simulink model "Sistema"  (R2023a)
settings: Solver=ode15s  StartTime=0.0  StopTime=10.0  MaxStep=1E-3  RelTol=1e-3
libraries: fl_lib x18, nesl_utility x9, ee_lib x3, slpidlib x2
settings Model: LastModifiedBy=alan_25
settings DataIOCC: SaveFormat=Array  ReturnWorkspaceOutputs=off  TimeSaveName=t
settings DebuggingCC: AlgebraicLoopMsg=none  ArtificialAlgebraicLoopMsg=none  ModelReferenceExtraNoncontSigs=none  OperatingPointInterfaceChecksumMismatchMsg=none
settings RTWCC: GPUComputeCapability=5.0

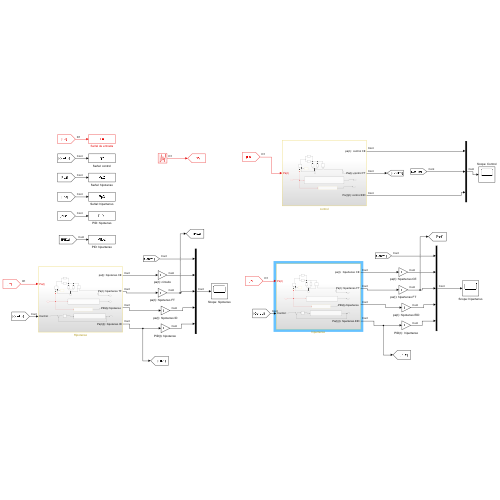
[thumbnail: Simulink's stored preview of the top-level diagram]
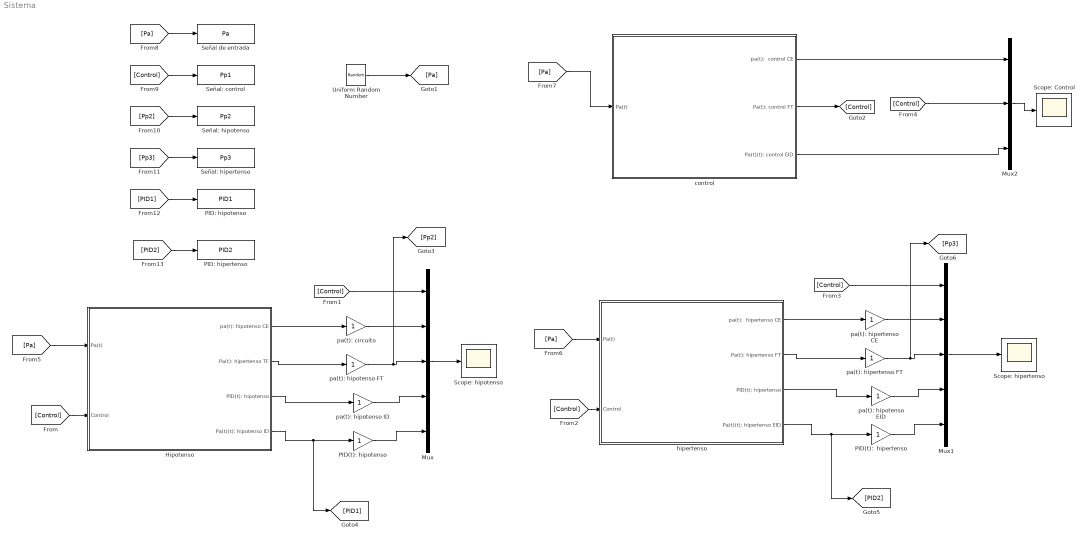
== system Sistema ==
  Hipotenso : Subsystem
  Mux : Mux  Inputs=5
  Mux1 : Mux  Inputs=5
  Mux2 : Mux  Inputs=3
  PID(t):  hipertenso : Gain
  "PID(t): hipotenso " : Gain
  PID: hipertenso : ToWorkspace  VariableName=PID2  SampleTime=-1
  PID: hipotenso : ToWorkspace  VariableName=PID1  SampleTime=-1
  Scope: Control : Scope
  Scope: hipertenso : Scope
  Scope: hipotenso : Scope
  Señal de entrada : ToWorkspace  VariableName=Pa  SampleTime=-1
  Señal: control : ToWorkspace  VariableName=Pp1  SampleTime=-1
  Señal: hipertenso : ToWorkspace  VariableName=Pp3  SampleTime=-1
  Señal: hipotenso : ToWorkspace  VariableName=Pp2  SampleTime=-1
  Uniform Random Number : UniformRandomNumber  Minimum=-0.2  Seed=106  SampleTime=0.5
  control : Subsystem
  hipertenso : Subsystem
  pa(t): circuito : Gain
  pa(t): hipertenso CE : Gain
  pa(t): hipertenso FT : Gain
  pa(t): hipotenso EID : Gain
  pa(t): hipotenso FT : Gain
  pa(t): hipotenso ID : Gain
  wires:
  Mux/1 -> Scope: hipotenso/1
  [Control] -> Hipotenso/2(Control)
  [Control] -> Mux/1
  Hipotenso/1(pa(t): hipotenso CE) -> pa(t): circuito/1
  pa(t): circuito/1 -> Mux/2
  "PID(t): hipotenso "/1 -> Mux/5
  Hipotenso/4(Pa(t)(t): hipotenso ID) -> [PID1], "PID(t): hipotenso "/1
  Hipotenso/3("PID(t): hipotenso ") -> pa(t): hipotenso ID/1
  pa(t): hipotenso ID/1 -> Mux/4
  pa(t): hipotenso FT/1 -> [Pp2], Mux/3
  Hipotenso/2(Pa(t): hipertenso TF) -> pa(t): hipotenso FT/1
  hipertenso/1(pa(t):  hipertenso CE) -> pa(t): hipertenso CE/1
  pa(t): hipertenso FT/1 -> [Pp3], Mux1/3
  hipertenso/2(Pa(t): hipertenso FT) -> pa(t): hipertenso FT/1
  pa(t): hipotenso EID/1 -> Mux1/4
  [Control] -> hipertenso/2(Control)
  Mux1/1 -> Scope: hipertenso/1
  [Control] -> Mux1/1
  pa(t): hipertenso CE/1 -> Mux1/2
  hipertenso/4(Pa(t)(t): hipertenso EID) -> [PID2], PID(t):  hipertenso/1
  PID(t):  hipertenso/1 -> Mux1/5
  hipertenso/3("PID(t): hipertenso ") -> pa(t): hipotenso EID/1
  Uniform Random Number/1 -> [Pa]
  [Pa] -> Hipotenso/1(Pa(t))
  [Pa] -> hipertenso/1(Pa(t))
  Mux2/1 -> Scope: Control/1
  [Pa] -> control/1(Pa(t))
  control/2(Pa(t): control FT) -> [Control]
  [Control] -> Mux2/2
  control/1(pa(t):  control CE) -> Mux2/1
  control/3(Pa(t)(t): control EID) -> Mux2/3
  [Pa] -> Señal de entrada/1
  [Control] -> Señal: control/1
  [Pp2] -> Señal: hipotenso/1
  [Pp3] -> Señal: hipertenso/1
  [PID1] -> PID: hipotenso/1
  [PID2] -> PID: hipertenso/1

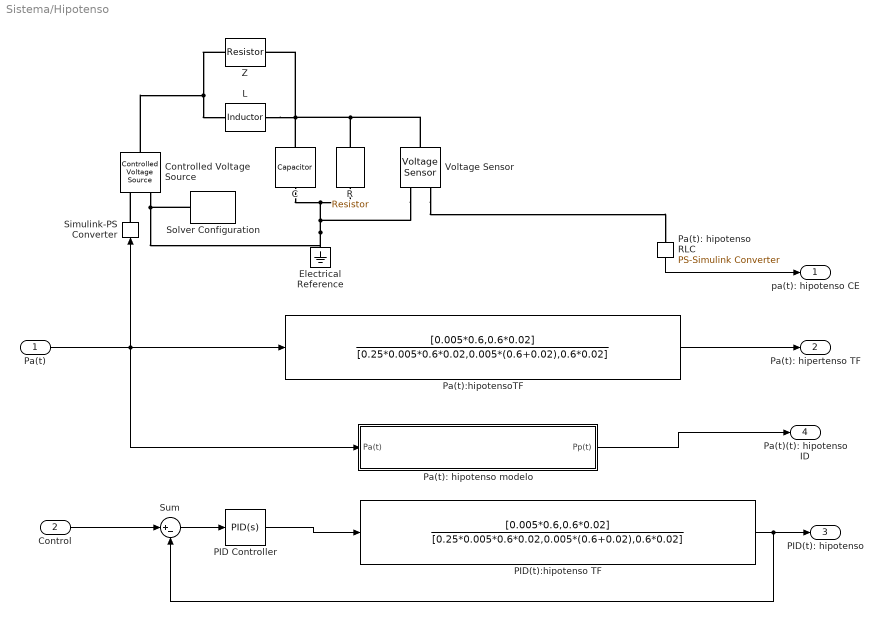
== system Sistema/Hipotenso ==
  Pa(t) : Inport
  Control : Inport  Port=2
  C : fl_lib/Electrical/Electrical Elements/Capacitor  c=0.25 F  r=1e-6 Ohm  g=0 1/Ohm  i_specify=off  i_priority=None  i=0 A  i_nominal_specify=off  i_nominal_unit=A  i_nominal_value=1  v_specify=off  v_priority=None  v=0 V  v_nominal_specify=off  v_nominal_unit=V  v_nominal_value=1  vc_specify=off  vc_priority=High  vc=0 V  vc_nominal_specify=off  vc_nominal_unit=V  vc_nominal_value=1
  Controlled Voltage Source : fl_lib/Electrical/Electrical Sources/Controlled Voltage Source
  Electrical Reference : fl_lib/Electrical/Electrical Elements/Electrical Reference
  L : ee_lib/Passive/Inductor  l=0.005 H  enable_L_tol=ee.enum.toleranceApplication.none  L_tol=20  tol_distribution=ee.enum.toleranceDistribution.uniform  nSigma=4  r=0 Ohm  g=1e-9 1/Ohm  enable_operating_limits=ee.enum.enable.no  operating_limit_action=ee.enum.passive.reportOpLim.warn  max_working_current=1 A  power_rating=1 W  enable_faults=ee.enum.enable.no  fault_action=simscape.enum.assert.action.none  lambdaPercent=50  k_faulted=0.9999  turnsShort=ee.enum.passive.inductor.turnsShortOption.no  openCct=ee.enum.enable.no  groundShort=ee.enum.passive.inductor.groundShortOption.no  groundShortG=0 1/Ohm  tau_fault=1e-3 s  fault_trigger=ee.enum.faults.faultTrigger.temporal  t_fault=1 s  max_permissible_voltage=100 V  n_fail_on_voltage=1  max_permissible_current=1 A  t_fail_on_current=1 s  i_L_specify=off  i_L_priority=High  i_L=0 A  i_L_nominal_specify=off  i_L_nominal_unit=A  i_L_nominal_value=1
  PID Controller : slpidlib/PID Controller  Controller=PID  Form=Parallel  TimeDomain=Continuous-time  UseExternalTs=off  SampleTime=-1  IntegratorMethod=Forward Euler  FilterMethod=Forward Euler  ControllerParametersSource=internal  P=1.49397900518606  I=352.000659394334  UseKiTs=off  D=0.00049119206492278  N=536.918505743178  UseFilter=on  TunerSelectOption=Transfer Function Based (PID Tuner App)  InitialConditionSource=internal  InitialConditionForIntegrator=0  InitialConditionForFilter=0  DifferentiatorICPrevScaledInput=0  ExternalReset=none  TrackingMode=off  Kt=1  LimitOutput=off  SatLimitsSource=internal  UpperSaturationLimit=inf  LowerSaturationLimit=-inf  LinearizeAsGain=on  AntiWindupMode=none  Kb=1  LimitIntegrator=off  UpperIntegratorSaturationLimit=inf  LowerIntegratorSaturationLimit=-inf  POutMin=[]  POutMax=[]  IOutMin=[]  IOutMax=[]  DOutMin=[]  DOutMax=[]  NOutMin=[]  NOutMax=[]  SumOutMin=[]  SumOutMax=[]  SaturationOutMin=[]  SaturationOutMax=[]  PParamMin=[]  PParamMax=[]  IParamMin=[]  IParamMax=[]  DParamMin=[]  DParamMax=[]  NParamMin=[]  NParamMax=[]  KbParamMin=[]  KbParamMax=[]  KtParamMin=[]  KtParamMax=[]  KbOutMin=[]  KbOutMax=[]  KtOutMin=[]  KtOutMax=[]  IntegratorOutMin=[]  IntegratorOutMax=[]  FilterOutMin=[]  FilterOutMax=[]  SumI1OutMin=[]  SumI1OutMax=[]  SumI2OutMin=[]  SumI2OutMax=[]  SumI3OutMin=[]  SumI3OutMax=[]  SumI4OutMin=[]  SumI4OutMax=[]  SumDOutMin=[]  SumDOutMax=[]  DifferentiatorOutMin=[]  DifferentiatorOutMax=[]  FilterDiffOutCoefMin=[]  FilterDiffOutCoefMax=[]  ReciprocalOutMin=[]  ReciprocalOutMax=[]  SumDenOutMin=[]  SumDenOutMax=[]  SumNumOutMin=[]  SumNumOutMax=[]  DivideOutMin=[]  DivideOutMax=[]  UdiffTsProdOutMin=[]  UdiffTsProdOutMax=[]  NTsProdOutMin=[]  NTsProdOutMax=[]  UintegralTsProdOutMin=[]  UintegralTsProdOutMax=[]  UngainTsProdOutMin=[]  UngainTsProdOutMax=[]  ClampingZeroOutDataTypeStr=Inherit: Inherit via back propagation  ClampingZeroOutMin=[]  ClampingZeroOutMax=[]  FilterDenConstantOutDataTypeStr=Inherit: Inherit via back propagation  FilterDenConstantOutMin=[]  FilterDenConstantOutMax=[]  PCopyOutDataTypeStr=Inherit: Inherit via back propagation  PCopyOutMin=[]  PCopyOutMax=[]  NCopyOutDataTypeStr=Inherit: Inherit via back propagation  NCopyOutMin=[]  NCopyOutMax=[]  IntegratorContinuousStateAttributes=''  IntegratorStateMustResolveToSignalObject=off  IntegratorRTWStateStorageClass=Auto  FilterContinuousStateAttributes=''  FilterStateMustResolveToSignalObject=off  FilterRTWStateStorageClass=Auto  ParallelPVariant=InternalParameters  IdealPVariant=Disabled  IVariant=InternalParameters  DVariant=InternalParameters  IntegratorVariant=Continuous  SatVariant=Disabled  AWVariant=Passthrough  PCopyVariant=Disabled  TRVariant=Disabled  FdbkBlocksVariant=Forward  IdealPFdbkVariant=Disabled  SatFdbkVariant=Disabled  DerivativeFilterVariant=ContFilter  NVariant=InternalParameters  NCopyVariant=Disabled  FilterICVariant=InternalICsFilter  IntegratorICVariant=InternalICs  ExternalResetVariant=Disabled  TRSumVariant=Passthrough  SumFdbkVariant=Disabled  SumVariant=Sum_PID  TsampFilterVariant=InternalTs  TsampNgainVariant=Passthrough  TsampIntegralVariant=Disabled_SignalSpec  ExternalSaturationOutDataTypeStr=Inherit: Same as second input
  PID(t):hipotenso TF : TransferFcn  Numerator=[0.005*0.6,0.6*0.02]  Denominator=[0.25*0.005*0.6*0.02,0.005*(0.6+0.02),0.6*0.02]
  Pa(t): hipotenso RLC : nesl_utility/PS-Simulink Converter  PhysicalDomain=network_engine_domain  SubClassName=ps_output  LeftPortType=input  RightPortType=output  PseudoPeriodic=off  Frequencies=[]  VectorFormat=1-D array  Unit=inherit  AffineConversion=off
  Pa(t): hipotenso modelo : Subsystem  TreatAsAtomicUnit=on
  Pa(t):hipotensoTF : TransferFcn  Numerator=[0.005*0.6,0.6*0.02]  Denominator=[0.25*0.005*0.6*0.02,0.005*(0.6+0.02),0.6*0.02]
  R : fl_lib/Electrical/Electrical Elements/Resistor  R=0.6 Ohm  i_specify=off  i_priority=None  i=0 A  i_nominal_specify=off  i_nominal_unit=A  i_nominal_value=1  v_specify=off  v_priority=None  v=0 V  v_nominal_specify=off  v_nominal_unit=V  v_nominal_value=1
  Simulink-PS Converter : nesl_utility/Simulink-PS Converter  PhysicalDomain=network_engine_domain  SubClassName=ps_input  LeftPortType=input  RightPortType=output  PseudoPeriodic=off  Frequencies=[]  NoiseDistribution=none  NoiseParameters=[]  Unit=1  AffineConversion=off  FilteringAndDerivatives=provide  SimscapeFilterOrder=1  InputFilterTimeConstant=0.001  UdotUserProvided=0
  Solver Configuration : nesl_utility/Solver Configuration  PhysicalDomain=network_engine_domain  SubClassName=solver  LeftPortType=input  RightPortType=generic  Tones=[]  Harmonics=[]  SimulateNoise=off  Profile=off  UseLocalSampling=off  EnableSwitchedLinearOptims=on  FrequencyDomain=off  UseCCode=off  RelTol=0.001  AbsTol=0.001  MinStep=1e-09  ToWorkspace=off  RevertToSquareIcSolve=off  NumHomotopyIterations=100  PhasorMode=off  PhasorModeNumHarmonics=1  ConsistencySolver=NEWTON_XTOL_AFTER_FTOL  IndexReductionMethod=DerivativeReplacement  DoDC=off  ResidualTolerance=1e-09  ConsistencyTolSource=GLOBAL  ConsistencyAbsTol=0.001  ConsistencyRelTol=0.001  ConsistencyTolFactor=0.001  UseLocalSolver=off  LocalSolverChoice=NE_BACKWARD_EULER_ADVANCER  ResolveIndetEquations=on  FunctionEvalNumThread=1  LocalSolverSampleTime=0.001  DoFixedCost=off  MaxNonlinIter=3  MaxModeIter=2  ComputeImpulses=off  ImpulseIterations=2  LinearAlgebra=auto  LinearAlgebraNumThread=0  EquationFormulation=NE_TIME_EF  DelaysMemoryBudget=1024  AutomaticFiltering=on  FilteringTimeConstant=0.001  PartitionStorageMethod=AS_NEEDED  PartitionMemoryBudget=1024  PartitionMethod=ROBUST
  Sum : Sum  Inputs=|+-
  Voltage Sensor : fl_lib/Electrical/Electrical Sensors/Voltage Sensor
  Z : fl_lib/Electrical/Electrical Elements/Resistor  R=0.02 Ohm  i_specify=off  i_priority=None  i=0 A  i_nominal_specify=off  i_nominal_unit=A  i_nominal_value=1  v_specify=off  v_priority=None  v=0 V  v_nominal_specify=off  v_nominal_unit=V  v_nominal_value=1
  pa(t): hipotenso CE : Outport
  Pa(t): hipertenso TF : Outport  Port=2
  "PID(t): hipotenso " : Outport  Port=3
  Pa(t)(t): hipotenso ID : Outport  Port=4
  wires:
  PID(t):hipotenso TF/1 -> "PID(t): hipotenso "/1, Sum/2
  Sum/1 -> PID Controller/1
  PID Controller/1 -> PID(t):hipotenso TF/1
  Pa(t):hipotensoTF/1 -> Pa(t): hipertenso TF/1
  Pa(t): hipotenso RLC/1 -> pa(t): hipotenso CE/1
  Pa(t)/1 -> Pa(t): hipotenso modelo/1(Pa(t)), Pa(t):hipotensoTF/1, Simulink-PS Converter/1
  Control/1 -> Sum/1
  Pa(t): hipotenso modelo/1(Pp(t)) -> Pa(t)(t): hipotenso ID/1
  connections:
  Voltage Sensor/RConn1 -- Pa(t): hipotenso RLC/LConn1
  L/LConn1 -- Voltage Sensor/LConn1 -- R/LConn1 -- C/LConn1 -- Z/RConn1
  Simulink-PS Converter/RConn1 -- Controlled Voltage Source/RConn1
  Z/LConn1 -- Controlled Voltage Source/LConn1 -- L/RConn1
  C/RConn1 -- Voltage Sensor/RConn2 -- Solver Configuration/RConn1 -- Controlled Voltage Source/RConn2 -- Electrical Reference/LConn1 -- R/RConn1

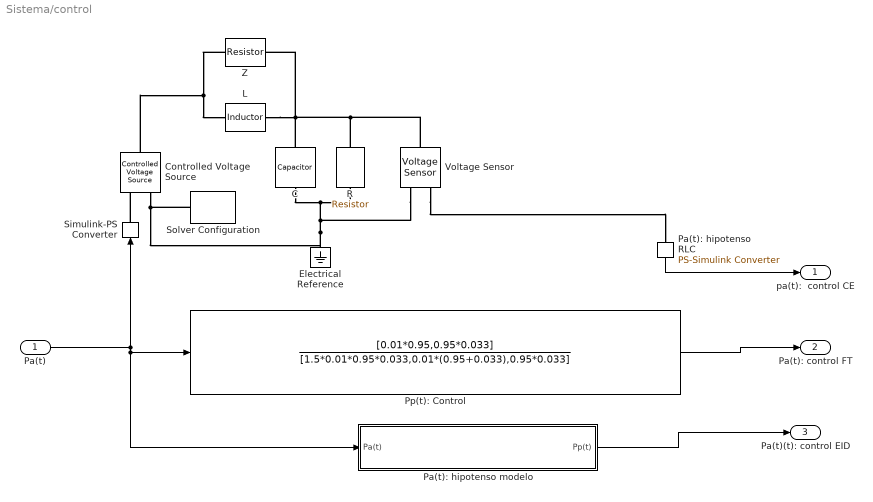
== system Sistema/control ==
  Pa(t) : Inport
  C : fl_lib/Electrical/Electrical Elements/Capacitor  c=1.5 F  r=1e-6 Ohm  g=0 1/Ohm  i_specify=off  i_priority=None  i=0 A  i_nominal_specify=off  i_nominal_unit=A  i_nominal_value=1  v_specify=off  v_priority=None  v=0 V  v_nominal_specify=off  v_nominal_unit=V  v_nominal_value=1  vc_specify=off  vc_priority=High  vc=0 V  vc_nominal_specify=off  vc_nominal_unit=V  vc_nominal_value=1
  Controlled Voltage Source : fl_lib/Electrical/Electrical Sources/Controlled Voltage Source
  Electrical Reference : fl_lib/Electrical/Electrical Elements/Electrical Reference
  L : ee_lib/Passive/Inductor  l=0.01 H  enable_L_tol=ee.enum.toleranceApplication.none  L_tol=20  tol_distribution=ee.enum.toleranceDistribution.uniform  nSigma=4  r=0 Ohm  g=1e-9 1/Ohm  enable_operating_limits=ee.enum.enable.no  operating_limit_action=ee.enum.passive.reportOpLim.warn  max_working_current=1 A  power_rating=1 W  enable_faults=ee.enum.enable.no  fault_action=simscape.enum.assert.action.none  lambdaPercent=50  k_faulted=0.9999  turnsShort=ee.enum.passive.inductor.turnsShortOption.no  openCct=ee.enum.enable.no  groundShort=ee.enum.passive.inductor.groundShortOption.no  groundShortG=0 1/Ohm  tau_fault=1e-3 s  fault_trigger=ee.enum.faults.faultTrigger.temporal  t_fault=1 s  max_permissible_voltage=100 V  n_fail_on_voltage=1  max_permissible_current=1 A  t_fail_on_current=1 s  i_L_specify=off  i_L_priority=High  i_L=0 A  i_L_nominal_specify=off  i_L_nominal_unit=A  i_L_nominal_value=1
  Pa(t): hipotenso RLC : nesl_utility/PS-Simulink Converter  PhysicalDomain=network_engine_domain  SubClassName=ps_output  LeftPortType=input  RightPortType=output  PseudoPeriodic=off  Frequencies=[]  VectorFormat=1-D array  Unit=inherit  AffineConversion=off
  Pa(t): hipotenso modelo : Subsystem  TreatAsAtomicUnit=on
  Pp(t): Control : TransferFcn  Numerator=[0.01*0.95,0.95*0.033]  Denominator=[1.5*0.01*0.95*0.033,0.01*(0.95+0.033),0.95*0.033]
  R : fl_lib/Electrical/Electrical Elements/Resistor  R=0.95 Ohm  i_specify=off  i_priority=None  i=0 A  i_nominal_specify=off  i_nominal_unit=A  i_nominal_value=1  v_specify=off  v_priority=None  v=0 V  v_nominal_specify=off  v_nominal_unit=V  v_nominal_value=1
  Simulink-PS Converter : nesl_utility/Simulink-PS Converter  PhysicalDomain=network_engine_domain  SubClassName=ps_input  LeftPortType=input  RightPortType=output  PseudoPeriodic=off  Frequencies=[]  NoiseDistribution=none  NoiseParameters=[]  Unit=1  AffineConversion=off  FilteringAndDerivatives=provide  SimscapeFilterOrder=1  InputFilterTimeConstant=0.001  UdotUserProvided=0
  Solver Configuration : nesl_utility/Solver Configuration  PhysicalDomain=network_engine_domain  SubClassName=solver  LeftPortType=input  RightPortType=generic  Tones=[]  Harmonics=[]  SimulateNoise=off  Profile=off  UseLocalSampling=off  EnableSwitchedLinearOptims=on  FrequencyDomain=off  UseCCode=off  RelTol=0.001  AbsTol=0.001  MinStep=1e-09  ToWorkspace=off  RevertToSquareIcSolve=off  NumHomotopyIterations=100  PhasorMode=off  PhasorModeNumHarmonics=1  ConsistencySolver=NEWTON_XTOL_AFTER_FTOL  IndexReductionMethod=DerivativeReplacement  DoDC=off  ResidualTolerance=1e-09  ConsistencyTolSource=GLOBAL  ConsistencyAbsTol=0.001  ConsistencyRelTol=0.001  ConsistencyTolFactor=0.001  UseLocalSolver=off  LocalSolverChoice=NE_BACKWARD_EULER_ADVANCER  ResolveIndetEquations=on  FunctionEvalNumThread=1  LocalSolverSampleTime=0.001  DoFixedCost=off  MaxNonlinIter=3  MaxModeIter=2  ComputeImpulses=off  ImpulseIterations=2  LinearAlgebra=auto  LinearAlgebraNumThread=0  EquationFormulation=NE_TIME_EF  DelaysMemoryBudget=1024  AutomaticFiltering=on  FilteringTimeConstant=0.001  PartitionStorageMethod=AS_NEEDED  PartitionMemoryBudget=1024  PartitionMethod=ROBUST
  Voltage Sensor : fl_lib/Electrical/Electrical Sensors/Voltage Sensor
  Z : fl_lib/Electrical/Electrical Elements/Resistor  R=0.033 Ohm  i_specify=off  i_priority=None  i=0 A  i_nominal_specify=off  i_nominal_unit=A  i_nominal_value=1  v_specify=off  v_priority=None  v=0 V  v_nominal_specify=off  v_nominal_unit=V  v_nominal_value=1
  pa(t):  control CE : Outport
  Pa(t): control FT : Outport  Port=2
  Pa(t)(t): control EID : Outport  Port=3
  wires:
  Pa(t): hipotenso RLC/1 -> pa(t):  control CE/1
  Pa(t)/1 -> Pp(t): Control/1, Pa(t): hipotenso modelo/1(Pa(t)), Simulink-PS Converter/1
  Pa(t): hipotenso modelo/1(Pp(t)) -> Pa(t)(t): control EID/1
  Pp(t): Control/1 -> Pa(t): control FT/1
  connections:
  Voltage Sensor/RConn1 -- Pa(t): hipotenso RLC/LConn1
  C/LConn1 -- Z/RConn1 -- L/LConn1 -- Voltage Sensor/LConn1 -- R/LConn1
  Simulink-PS Converter/RConn1 -- Controlled Voltage Source/RConn1
  Z/LConn1 -- L/RConn1 -- Controlled Voltage Source/LConn1
  Electrical Reference/LConn1 -- Voltage Sensor/RConn2 -- C/RConn1 -- R/RConn1 -- Solver Configuration/RConn1 -- Controlled Voltage Source/RConn2

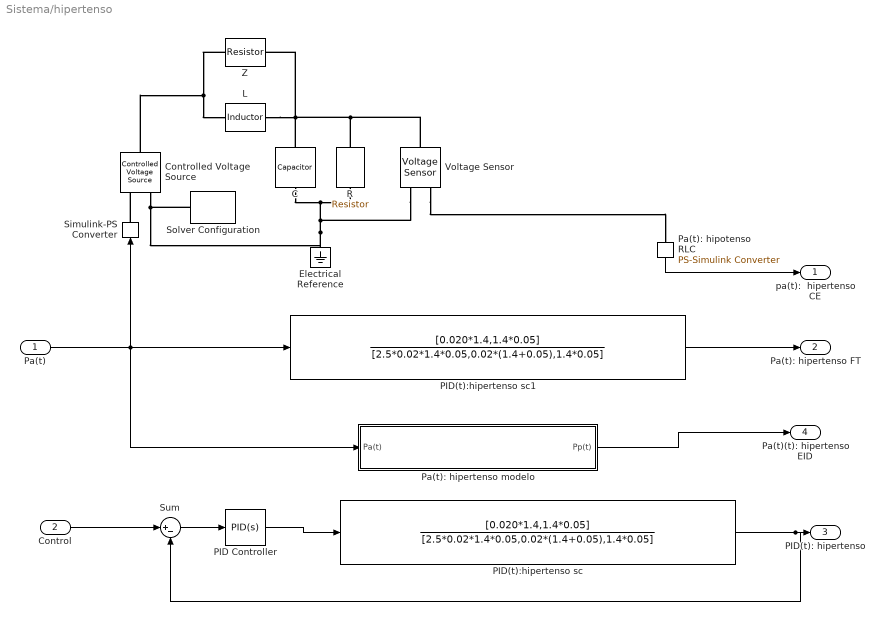
== system Sistema/hipertenso ==
  Pa(t) : Inport
  Control : Inport  Port=2
  C : fl_lib/Electrical/Electrical Elements/Capacitor  c=2.5 F  r=1e-6 Ohm  g=0 1/Ohm  i_specify=off  i_priority=None  i=0 A  i_nominal_specify=off  i_nominal_unit=A  i_nominal_value=1  v_specify=off  v_priority=None  v=0 V  v_nominal_specify=off  v_nominal_unit=V  v_nominal_value=1  vc_specify=off  vc_priority=High  vc=0 V  vc_nominal_specify=off  vc_nominal_unit=V  vc_nominal_value=1
  Controlled Voltage Source : fl_lib/Electrical/Electrical Sources/Controlled Voltage Source
  Electrical Reference : fl_lib/Electrical/Electrical Elements/Electrical Reference
  L : ee_lib/Passive/Inductor  l=0.02 H  enable_L_tol=ee.enum.toleranceApplication.none  L_tol=20  tol_distribution=ee.enum.toleranceDistribution.uniform  nSigma=4  r=0 Ohm  g=1e-9 1/Ohm  enable_operating_limits=ee.enum.enable.no  operating_limit_action=ee.enum.passive.reportOpLim.warn  max_working_current=1 A  power_rating=1 W  enable_faults=ee.enum.enable.no  fault_action=simscape.enum.assert.action.none  lambdaPercent=50  k_faulted=0.9999  turnsShort=ee.enum.passive.inductor.turnsShortOption.no  openCct=ee.enum.enable.no  groundShort=ee.enum.passive.inductor.groundShortOption.no  groundShortG=0 1/Ohm  tau_fault=1e-3 s  fault_trigger=ee.enum.faults.faultTrigger.temporal  t_fault=1 s  max_permissible_voltage=100 V  n_fail_on_voltage=1  max_permissible_current=1 A  t_fail_on_current=1 s  i_L_specify=off  i_L_priority=High  i_L=0 A  i_L_nominal_specify=off  i_L_nominal_unit=A  i_L_nominal_value=1
  PID Controller : slpidlib/PID Controller  Controller=PID  Form=Parallel  TimeDomain=Continuous-time  UseExternalTs=off  SampleTime=-1  IntegratorMethod=Forward Euler  FilterMethod=Forward Euler  ControllerParametersSource=internal  P=12.7154893348189  I=363.894411463659  UseKiTs=off  D=0.0343454696960019  N=139.99351585004  UseFilter=on  TunerSelectOption=Transfer Function Based (PID Tuner App)  InitialConditionSource=internal  InitialConditionForIntegrator=0  InitialConditionForFilter=0  DifferentiatorICPrevScaledInput=0  ExternalReset=none  TrackingMode=off  Kt=1  LimitOutput=off  SatLimitsSource=internal  UpperSaturationLimit=inf  LowerSaturationLimit=-inf  LinearizeAsGain=on  AntiWindupMode=none  Kb=1  LimitIntegrator=off  UpperIntegratorSaturationLimit=inf  LowerIntegratorSaturationLimit=-inf  POutMin=[]  POutMax=[]  IOutMin=[]  IOutMax=[]  DOutMin=[]  DOutMax=[]  NOutMin=[]  NOutMax=[]  SumOutMin=[]  SumOutMax=[]  SaturationOutMin=[]  SaturationOutMax=[]  PParamMin=[]  PParamMax=[]  IParamMin=[]  IParamMax=[]  DParamMin=[]  DParamMax=[]  NParamMin=[]  NParamMax=[]  KbParamMin=[]  KbParamMax=[]  KtParamMin=[]  KtParamMax=[]  KbOutMin=[]  KbOutMax=[]  KtOutMin=[]  KtOutMax=[]  IntegratorOutMin=[]  IntegratorOutMax=[]  FilterOutMin=[]  FilterOutMax=[]  SumI1OutMin=[]  SumI1OutMax=[]  SumI2OutMin=[]  SumI2OutMax=[]  SumI3OutMin=[]  SumI3OutMax=[]  SumI4OutMin=[]  SumI4OutMax=[]  SumDOutMin=[]  SumDOutMax=[]  DifferentiatorOutMin=[]  DifferentiatorOutMax=[]  FilterDiffOutCoefMin=[]  FilterDiffOutCoefMax=[]  ReciprocalOutMin=[]  ReciprocalOutMax=[]  SumDenOutMin=[]  SumDenOutMax=[]  SumNumOutMin=[]  SumNumOutMax=[]  DivideOutMin=[]  DivideOutMax=[]  UdiffTsProdOutMin=[]  UdiffTsProdOutMax=[]  NTsProdOutMin=[]  NTsProdOutMax=[]  UintegralTsProdOutMin=[]  UintegralTsProdOutMax=[]  UngainTsProdOutMin=[]  UngainTsProdOutMax=[]  ClampingZeroOutDataTypeStr=Inherit: Inherit via back propagation  ClampingZeroOutMin=[]  ClampingZeroOutMax=[]  FilterDenConstantOutDataTypeStr=Inherit: Inherit via back propagation  FilterDenConstantOutMin=[]  FilterDenConstantOutMax=[]  PCopyOutDataTypeStr=Inherit: Inherit via back propagation  PCopyOutMin=[]  PCopyOutMax=[]  NCopyOutDataTypeStr=Inherit: Inherit via back propagation  NCopyOutMin=[]  NCopyOutMax=[]  IntegratorContinuousStateAttributes=''  IntegratorStateMustResolveToSignalObject=off  IntegratorRTWStateStorageClass=Auto  FilterContinuousStateAttributes=''  FilterStateMustResolveToSignalObject=off  FilterRTWStateStorageClass=Auto  ParallelPVariant=InternalParameters  IdealPVariant=Disabled  IVariant=InternalParameters  DVariant=InternalParameters  IntegratorVariant=Continuous  SatVariant=Disabled  AWVariant=Passthrough  PCopyVariant=Disabled  TRVariant=Disabled  FdbkBlocksVariant=Forward  IdealPFdbkVariant=Disabled  SatFdbkVariant=Disabled  DerivativeFilterVariant=ContFilter  NVariant=InternalParameters  NCopyVariant=Disabled  FilterICVariant=InternalICsFilter  IntegratorICVariant=InternalICs  ExternalResetVariant=Disabled  TRSumVariant=Passthrough  SumFdbkVariant=Disabled  SumVariant=Sum_PID  TsampFilterVariant=InternalTs  TsampNgainVariant=Passthrough  TsampIntegralVariant=Disabled_SignalSpec  ExternalSaturationOutDataTypeStr=Inherit: Same as second input
  PID(t):hipertenso sc : TransferFcn  Numerator=[0.020*1.4,1.4*0.05]  Denominator=[2.5*0.02*1.4*0.05,0.02*(1.4+0.05),1.4*0.05]
  PID(t):hipertenso sc1 : TransferFcn  Numerator=[0.020*1.4,1.4*0.05]  Denominator=[2.5*0.02*1.4*0.05,0.02*(1.4+0.05),1.4*0.05]
  Pa(t): hipertenso modelo : Subsystem  TreatAsAtomicUnit=on
  Pa(t): hipotenso RLC : nesl_utility/PS-Simulink Converter  PhysicalDomain=network_engine_domain  SubClassName=ps_output  LeftPortType=input  RightPortType=output  PseudoPeriodic=off  Frequencies=[]  VectorFormat=1-D array  Unit=inherit  AffineConversion=off
  R : fl_lib/Electrical/Electrical Elements/Resistor  R=1.4 Ohm  i_specify=off  i_priority=None  i=0 A  i_nominal_specify=off  i_nominal_unit=A  i_nominal_value=1  v_specify=off  v_priority=None  v=0 V  v_nominal_specify=off  v_nominal_unit=V  v_nominal_value=1
  Simulink-PS Converter : nesl_utility/Simulink-PS Converter  PhysicalDomain=network_engine_domain  SubClassName=ps_input  LeftPortType=input  RightPortType=output  PseudoPeriodic=off  Frequencies=[]  NoiseDistribution=none  NoiseParameters=[]  Unit=1  AffineConversion=off  FilteringAndDerivatives=provide  SimscapeFilterOrder=1  InputFilterTimeConstant=0.001  UdotUserProvided=0
  Solver Configuration : nesl_utility/Solver Configuration  PhysicalDomain=network_engine_domain  SubClassName=solver  LeftPortType=input  RightPortType=generic  Tones=[]  Harmonics=[]  SimulateNoise=off  Profile=off  UseLocalSampling=off  EnableSwitchedLinearOptims=on  FrequencyDomain=off  UseCCode=off  RelTol=0.001  AbsTol=0.001  MinStep=1e-09  ToWorkspace=off  RevertToSquareIcSolve=off  NumHomotopyIterations=100  PhasorMode=off  PhasorModeNumHarmonics=1  ConsistencySolver=NEWTON_XTOL_AFTER_FTOL  IndexReductionMethod=DerivativeReplacement  DoDC=off  ResidualTolerance=1e-09  ConsistencyTolSource=GLOBAL  ConsistencyAbsTol=0.001  ConsistencyRelTol=0.001  ConsistencyTolFactor=0.001  UseLocalSolver=off  LocalSolverChoice=NE_BACKWARD_EULER_ADVANCER  ResolveIndetEquations=on  FunctionEvalNumThread=1  LocalSolverSampleTime=0.001  DoFixedCost=off  MaxNonlinIter=3  MaxModeIter=2  ComputeImpulses=off  ImpulseIterations=2  LinearAlgebra=auto  LinearAlgebraNumThread=0  EquationFormulation=NE_TIME_EF  DelaysMemoryBudget=1024  AutomaticFiltering=on  FilteringTimeConstant=0.001  PartitionStorageMethod=AS_NEEDED  PartitionMemoryBudget=1024  PartitionMethod=ROBUST
  Sum : Sum  Inputs=|+-
  Voltage Sensor : fl_lib/Electrical/Electrical Sensors/Voltage Sensor
  Z : fl_lib/Electrical/Electrical Elements/Resistor  R=0.05 Ohm  i_specify=off  i_priority=None  i=0 A  i_nominal_specify=off  i_nominal_unit=A  i_nominal_value=1  v_specify=off  v_priority=None  v=0 V  v_nominal_specify=off  v_nominal_unit=V  v_nominal_value=1
  pa(t):  hipertenso CE : Outport
  Pa(t): hipertenso FT : Outport  Port=2
  "PID(t): hipertenso " : Outport  Port=3
  Pa(t)(t): hipertenso EID : Outport  Port=4
  wires:
  PID(t):hipertenso sc/1 -> "PID(t): hipertenso "/1, Sum/2
  Sum/1 -> PID Controller/1
  PID(t):hipertenso sc1/1 -> Pa(t): hipertenso FT/1
  Pa(t): hipotenso RLC/1 -> pa(t):  hipertenso CE/1
  Pa(t)/1 -> PID(t):hipertenso sc1/1, Pa(t): hipertenso modelo/1(Pa(t)), Simulink-PS Converter/1
  Control/1 -> Sum/1
  Pa(t): hipertenso modelo/1(Pp(t)) -> Pa(t)(t): hipertenso EID/1
  PID Controller/1 -> PID(t):hipertenso sc/1
  connections:
  Voltage Sensor/RConn1 -- Pa(t): hipotenso RLC/LConn1
  C/LConn1 -- Z/RConn1 -- L/LConn1 -- Voltage Sensor/LConn1 -- R/LConn1
  Simulink-PS Converter/RConn1 -- Controlled Voltage Source/RConn1
  Z/LConn1 -- L/RConn1 -- Controlled Voltage Source/LConn1
  Electrical Reference/LConn1 -- Voltage Sensor/RConn2 -- C/RConn1 -- R/RConn1 -- Solver Configuration/RConn1 -- Controlled Voltage Source/RConn2

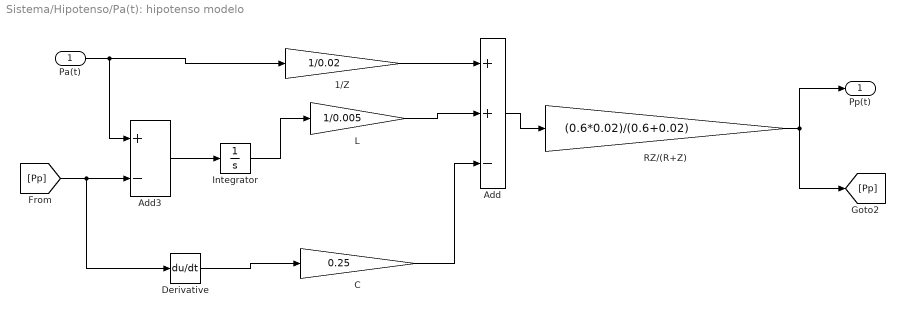
== system Sistema/Hipotenso/Pa(t): hipotenso modelo ==
  Pa(t) : Inport
  1/Z : Gain  Gain=1/0.02
  Add : Sum  Inputs=++-
  Add3 : Sum  Inputs=+-
  C : Gain  Gain=0.25
  Derivative : Derivative
  Integrator : Integrator
  L : Gain  Gain=1/0.005
  RZ/(R+Z) : Gain  Gain=(0.6*0.02)/(0.6+0.02)
  Pp(t) : Outport
  wires:
  Add/1 -> RZ/(R+Z)/1
  RZ/(R+Z)/1 -> Pp(t)/1, [Pp]
  Pa(t)/1 -> Add3/1, 1/Z/1
  Add3/1 -> Integrator/1
  Integrator/1 -> L/1
  1/Z/1 -> Add/1
  L/1 -> Add/2
  C/1 -> Add/3
  [Pp] -> Derivative/1, Add3/2
  Derivative/1 -> C/1

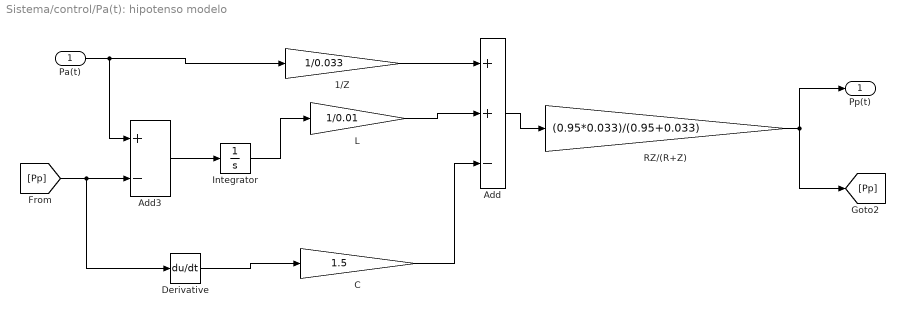
== system Sistema/control/Pa(t): hipotenso modelo ==
  Pa(t) : Inport
  1/Z : Gain  Gain=1/0.033
  Add : Sum  Inputs=++-
  Add3 : Sum  Inputs=+-
  C : Gain  Gain=1.5
  Derivative : Derivative
  Integrator : Integrator
  L : Gain  Gain=1/0.01
  RZ/(R+Z) : Gain  Gain=(0.95*0.033)/(0.95+0.033)
  Pp(t) : Outport
  wires:
  Add/1 -> RZ/(R+Z)/1
  RZ/(R+Z)/1 -> Pp(t)/1, [Pp]
  Pa(t)/1 -> Add3/1, 1/Z/1
  Add3/1 -> Integrator/1
  Integrator/1 -> L/1
  1/Z/1 -> Add/1
  L/1 -> Add/2
  C/1 -> Add/3
  [Pp] -> Derivative/1, Add3/2
  Derivative/1 -> C/1

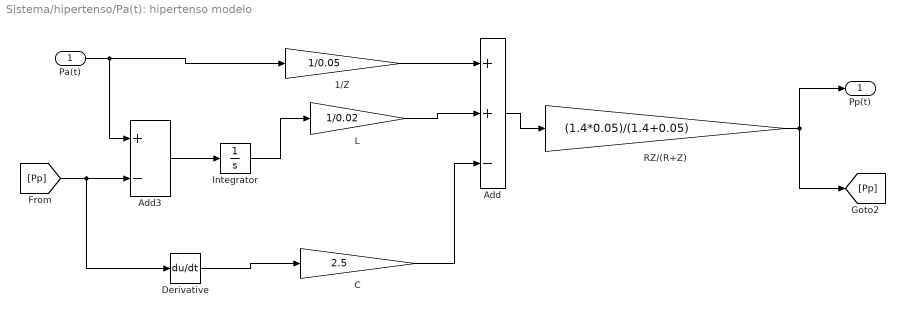
== system Sistema/hipertenso/Pa(t): hipertenso modelo ==
  Pa(t) : Inport
  1/Z : Gain  Gain=1/0.05
  Add : Sum  Inputs=++-
  Add3 : Sum  Inputs=+-
  C : Gain  Gain=2.5
  Derivative : Derivative
  Integrator : Integrator
  L : Gain  Gain=1/0.02
  RZ/(R+Z) : Gain  Gain=(1.4*0.05)/(1.4+0.05)
  Pp(t) : Outport
  wires:
  Add/1 -> RZ/(R+Z)/1
  RZ/(R+Z)/1 -> Pp(t)/1, [Pp]
  Pa(t)/1 -> Add3/1, 1/Z/1
  Add3/1 -> Integrator/1
  Integrator/1 -> L/1
  1/Z/1 -> Add/1
  L/1 -> Add/2
  C/1 -> Add/3
  [Pp] -> Derivative/1, Add3/2
  Derivative/1 -> C/1
